simulink model "amalifuzzypid"  (R2021a)
settings: Solver=FixedStepAuto  StartTime=0.0  StopTime=20  RelTol=1e-2  EnableMultiTasking=on
InitFcn:
  | Ts=0.01;
  | 
  | Kpmin1 = 0.1;
  | Kpmax1 = 5;
  | Kdmin1 = 0;
  | Kdmax1 = 2;
undefined symbols (not defined in the file): DiscIntNeverNeededParam
libraries: raspberrypiCommlib x6, pid_lib x4, raspberrypiBasiclib x4, fuzblock x2
settings Model: Creator=pouria  LastModifiedBy=pouria
settings SolverCC: AlgebraicLoopSolver=TrustRegion  PositivePriorityOrder=on
settings DataIOCC: LimitDataPoints=on  SaveFormat=Array  ReturnWorkspaceOutputs=off
settings OptimizationCC: EnhancedBackFolding=on  PassReuseOutputArgsAs=Individual arguments  ZeroExternalMemoryAtStartup=off  ZeroInternalMemoryAtStartup=off  MaxStackSize=64  OptimizeBlockOrder=speed  DifferentSizesBufferReuse=on  OptimizationCustomize=off  EfficientTunableParamExpr=on
settings DebuggingCC: ParameterTunabilityLossMsg=error  SFUnexpectedBacktrackingDiag=warning  SFNoUnconditionalDefaultTransitionDiag=warning  SFExecutionAtInitializationDiag=none  SFMachineParentedDataDiag=warning  ArithmeticOperatorsInVariantConditions=warning
settings HardwareCC: ProdBitPerPointer=32  ProdBitPerSizeT=32  ProdBitPerPtrDiffT=32  ProdLargestAtomicInteger=Long  ProdLargestAtomicFloat=Double  ProdWordSize=32  ProdLongLongMode=on  ProdHWDeviceType=ARM Compatible->ARM Cortex
settings ModelReferenceCC: PropagateSignalLabelsOutOfModel=off
settings SFSimCC: SimUseLocalCustomCode=off  CustomCodeUndefinedFunction=UseInterfaceOnly
settings RTWCC: SystemTargetFile=ert.tlc  HardwareBoard=Raspberry Pi  TLCOptions="-aInlineSetEventsForThisBaseRateFcn=TLC_FALSE -aSuppressMultiTaskScheduler=TLC_FALSE  -aRateBasedStepFcn=0"  TemplateMakefile=ert_default_tmf  RTWUseLocalCustomCode=off  Toolchain=GNU GCC Embedded Linux  BuildConfiguration=Faster Runs
settings CodeAppCC: ForceParamTrailComments=on  IgnoreCustomStorageClasses=off  OperatorAnnotations=on  SimulinkDataObjDesc=on  SFDataObjDesc=on  InsertBlockDesc=on
settings ERTTargetCC: SupportContinuousTime=on  SupportVariableSizeSignals=on  ExtModeTransport=2  ExtModeStaticAlloc=on  ExtModeMexFile=ext_xcp  ExtModeIntrfLevel=Level2 - Open
settings ConfigComp: CovMetricSettings=dw  CovSaveCumulativeToWorkspaceVar=on  CovSaveSingleToWorkspaceVar=on  CovExternalEMLEnable=off  CovSFcnEnable=off

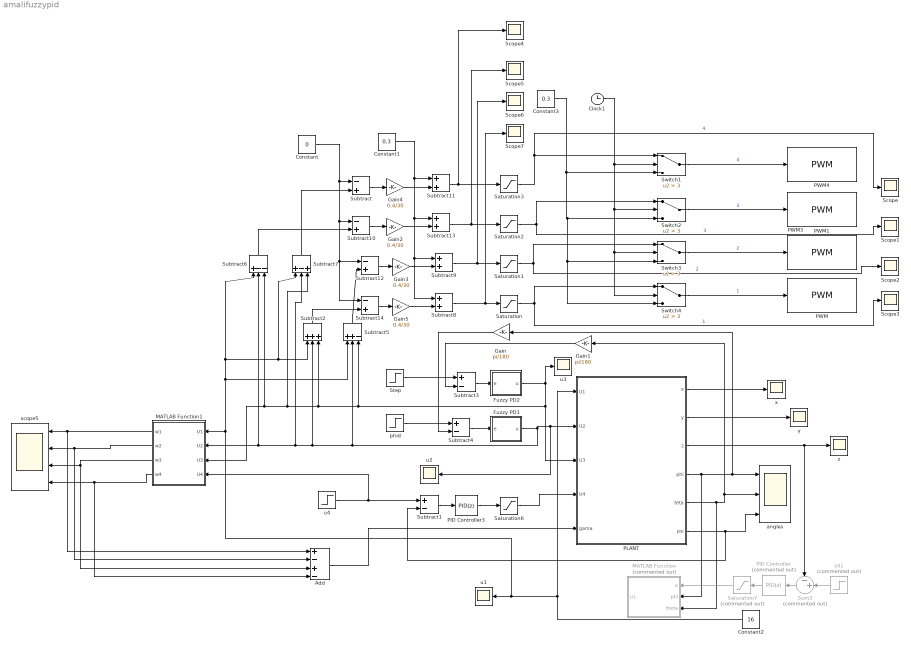
== system amalifuzzypid ==
  Add : Sum  Inputs=+-+-
  Clock1 : Clock
  Constant : Constant  Value=0  SampleTime=Ts
  Constant1 : Constant  Value=0.3  SampleTime=Ts
  Constant2 : Constant  Value=16  SampleTime=Ts
  Constant3 : Constant  Value=0.3  SampleTime=Ts
  Fuzzy PD1 : Subsystem
  Fuzzy PD2 : Subsystem
  Gain : Gain  Gain=pi/180
  Gain1 : Gain  Gain=pi/180
  Gain{2..5} (4 alike) : Gain  Gain=0.4/30
  MATLAB Function : MATLAB Function  Commented=on  TreatAsAtomicUnit=on
  MATLAB Function1 : MATLAB Function  TreatAsAtomicUnit=on
  PID Controller : pid_lib/PID Controller  Commented=on  Controller=PID  Form=Parallel  TimeDomain=Discrete-time  UseExternalTs=off  SampleTime=0.01  IntegratorMethod=Forward Euler  FilterMethod=Forward Euler  ControllerParametersSource=internal  P=5  I=2  D=15  UseFilter=on  N=20  TunerSelectOption=Transfer Function Based (PID Tuner App)  InitialConditionSource=internal  InitialConditionForIntegrator=0  InitialConditionForFilter=0  DifferentiatorICPrevScaledInput=0  ExternalReset=none  TrackingMode=off  Kt=1  LimitOutput=off  SatLimitsSource=internal  UpperSaturationLimit=inf  LowerSaturationLimit=-inf  LinearizeAsGain=on  AntiWindupMode=none  Kb=1  POutMin=[]  POutMax=[]  IOutMin=[]  IOutMax=[]  DOutMin=[]  DOutMax=[]  NOutMin=[]  NOutMax=[]  SumOutMin=[]  SumOutMax=[]  SaturationOutMin=[]  SaturationOutMax=[]  PParamMin=[]  PParamMax=[]  IParamMin=[]  IParamMax=[]  DParamMin=[]  DParamMax=[]  NParamMin=[]  NParamMax=[]  KbParamMin=[]  KbParamMax=[]  KtParamMin=[]  KtParamMax=[]  KbOutMin=[]  KbOutMax=[]  KtOutMin=[]  KtOutMax=[]  IntegratorOutMin=[]  IntegratorOutMax=[]  FilterOutMin=[]  FilterOutMax=[]  SumI1OutMin=[]  SumI1OutMax=[]  SumI2OutMin=[]  SumI2OutMax=[]  SumI3OutMin=[]  SumI3OutMax=[]  SumI4OutMin=[]  SumI4OutMax=[]  SumDOutMin=[]  SumDOutMax=[]  DifferentiatorOutMin=[]  DifferentiatorOutMax=[]  FilterDiffOutCoefMin=[]  FilterDiffOutCoefMax=[]  ReciprocalOutMin=[]  ReciprocalOutMax=[]  SumDenOutMin=[]  SumDenOutMax=[]  SumNumOutMin=[]  SumNumOutMax=[]  DivideOutMin=[]  DivideOutMax=[]  UdiffTsProdOutMin=[]  UdiffTsProdOutMax=[]  NTsProdOutMin=[]  NTsProdOutMax=[]  UintegralTsProdOutMin=[]  UintegralTsProdOutMax=[]  UngainTsProdOutMin=[]  UngainTsProdOutMax=[]  IntegratorContinuousStateAttributes=''  IntegratorStateMustResolveToSignalObject=off  IntegratorRTWStateStorageClass=Auto  FilterContinuousStateAttributes=''  FilterStateMustResolveToSignalObject=off  FilterRTWStateStorageClass=Auto  ParallelPVariant=InternalParameters  IdealPVariant=Disabled  IVariant=InternalParameters  DVariant=InternalParameters  IntegratorVariant=Discrete  SatVariant=Disabled  AWVariant=Passthrough  PCopyVariant=Disabled  TRVariant=Disabled  FdbkBlocksVariant=Forward  IdealPFdbkVariant=Disabled  SatFdbkVariant=Disabled  DerivativeFilterVariant=ForwardEulerFilter  NVariant=InternalParameters  NCopyVariant=Disabled  FilterICVariant=InternalICsFilter  IntegratorICVariant=InternalICs  ExternalResetVariant=Disabled  TRSumVariant=Passthrough  SumFdbkVariant=Disabled  SumVariant=Sum_PID  TsampFilterVariant=InternalTs  TsampNgainVariant=Passthrough  TsampIntegralVariant=Passthrough  ExternalSaturationOutDataTypeStr=Inherit: Same as second input
  PID Controller3 : pid_lib/PID Controller  Controller=PID  Form=Parallel  TimeDomain=Discrete-time  UseExternalTs=off  SampleTime=Ts  IntegratorMethod=Forward Euler  FilterMethod=Forward Euler  ControllerParametersSource=internal  P=0  I=0  D=0  UseFilter=on  N=20  TunerSelectOption=Transfer Function Based (PID Tuner App)  InitialConditionSource=internal  InitialConditionForIntegrator=0  InitialConditionForFilter=0  DifferentiatorICPrevScaledInput=0  ExternalReset=none  TrackingMode=off  Kt=1  LimitOutput=off  SatLimitsSource=internal  UpperSaturationLimit=inf  LowerSaturationLimit=-inf  LinearizeAsGain=on  AntiWindupMode=none  Kb=1  POutMin=[]  POutMax=[]  IOutMin=[]  IOutMax=[]  DOutMin=[]  DOutMax=[]  NOutMin=[]  NOutMax=[]  SumOutMin=[]  SumOutMax=[]  SaturationOutMin=[]  SaturationOutMax=[]  PParamMin=[]  PParamMax=[]  IParamMin=[]  IParamMax=[]  DParamMin=[]  DParamMax=[]  NParamMin=[]  NParamMax=[]  KbParamMin=[]  KbParamMax=[]  KtParamMin=[]  KtParamMax=[]  KbOutMin=[]  KbOutMax=[]  KtOutMin=[]  KtOutMax=[]  IntegratorOutMin=[]  IntegratorOutMax=[]  FilterOutMin=[]  FilterOutMax=[]  SumI1OutMin=[]  SumI1OutMax=[]  SumI2OutMin=[]  SumI2OutMax=[]  SumI3OutMin=[]  SumI3OutMax=[]  SumI4OutMin=[]  SumI4OutMax=[]  SumDOutMin=[]  SumDOutMax=[]  DifferentiatorOutMin=[]  DifferentiatorOutMax=[]  FilterDiffOutCoefMin=[]  FilterDiffOutCoefMax=[]  ReciprocalOutMin=[]  ReciprocalOutMax=[]  SumDenOutMin=[]  SumDenOutMax=[]  SumNumOutMin=[]  SumNumOutMax=[]  DivideOutMin=[]  DivideOutMax=[]  UdiffTsProdOutMin=[]  UdiffTsProdOutMax=[]  NTsProdOutMin=[]  NTsProdOutMax=[]  UintegralTsProdOutMin=[]  UintegralTsProdOutMax=[]  UngainTsProdOutMin=[]  UngainTsProdOutMax=[]  IntegratorContinuousStateAttributes=''  IntegratorStateMustResolveToSignalObject=off  IntegratorRTWStateStorageClass=Auto  FilterContinuousStateAttributes=''  FilterStateMustResolveToSignalObject=off  FilterRTWStateStorageClass=Auto  ParallelPVariant=InternalParameters  IdealPVariant=Disabled  IVariant=InternalParameters  DVariant=InternalParameters  IntegratorVariant=Discrete  SatVariant=Disabled  AWVariant=Passthrough  PCopyVariant=Disabled  TRVariant=Disabled  FdbkBlocksVariant=Forward  IdealPFdbkVariant=Disabled  SatFdbkVariant=Disabled  DerivativeFilterVariant=ForwardEulerFilter  NVariant=InternalParameters  NCopyVariant=Disabled  FilterICVariant=InternalICsFilter  IntegratorICVariant=InternalICs  ExternalResetVariant=Disabled  TRSumVariant=Passthrough  SumFdbkVariant=Disabled  SumVariant=Sum_PID  TsampFilterVariant=InternalTs  TsampNgainVariant=Passthrough  TsampIntegralVariant=Passthrough  ExternalSaturationOutDataTypeStr=Inherit: Same as second input
  PLANT : Subsystem
  PWM : raspberrypiBasiclib/PWM  board=Pi 3 Model B+  Pin_=21  Frequency=400  blockPlatform=Raspberry Pi
      settings: SourceProductBaseCode=RASPPI
  PWM1 : raspberrypiBasiclib/PWM  board=Pi 3 Model B+  Pin_=20  Frequency=400  blockPlatform=Raspberry Pi
      settings: SourceProductBaseCode=RASPPI
  PWM3 : raspberrypiBasiclib/PWM  board=Pi 3 Model B+  Pin_=16  Frequency=400  blockPlatform=Raspberry Pi
      settings: SourceProductBaseCode=RASPPI
  PWM4 : raspberrypiBasiclib/PWM  board=Pi 3 Model B+  Pin_=19  Frequency=400  blockPlatform=Raspberry Pi
      settings: SourceProductBaseCode=RASPPI
  Saturation{,1..3} (4 alike) : Saturate  UpperLimit=0.63  LowerLimit=0.3
  Saturation6 : Saturate
  Saturation7 : Saturate  Commented=on  UpperLimit=10  LowerLimit=-10
  Scope{,1..7} (8 alike) : Scope
  Step : Step  Time=0  After=0  SampleTime=0
  Subtract{,10,12,14} (4 alike) : Sum  Inputs=-+
  Subtract1 : Sum  Inputs=+-
  Subtract{8..9,11,13} (4 alike) : Sum
  Subtract2 : Sum  Inputs=+++
  Subtract3 : Sum  Inputs=+-
  Subtract4 : Sum  Inputs=+-
  Subtract5 : Sum  Inputs=++-
  Subtract6 : Sum  Inputs=+--
  Subtract7 : Sum  Inputs=+-+
  Sum2 : Sum  Commented=on  Inputs=-+|
  Switch{1..4} (4 alike) : Switch  Criteria=u2 > Threshold  Threshold=3
  angles : Scope  NumInputPorts=3
  phid : Step  Time=0  After=0  SampleTime=Ts
  scope5 : Scope  NumInputPorts=4
  u1 : Scope
  u2 : Scope
  u3 : Scope
  u4 : Step  Time=0  After=0  SampleTime=Ts
  x : Scope
  y : Scope
  z : Scope
  zd1 : Step  Commented=on  Time=0  After=0  SampleTime=0
  wires:
  PLANT/6(psi) -> angles/3, Subtract1/2
  PLANT/1(x) -> x/1
  PLANT/2(y) -> y/1
  Subtract4/1 -> Fuzzy PD1/1(e)
  Subtract3/1 -> Fuzzy PD2/1(e)
  Add/1 -> PLANT/5(gama)
  MATLAB Function1/1(w1) -> Add/1, scope5/1
  MATLAB Function1/3(w3) -> Add/3, scope5/3
  MATLAB Function1/4(w4) -> scope5/4, Add/4
  phid/1 -> Subtract4/1
  u4/1 -> MATLAB Function1/4(U4), Subtract1/1
  Subtract1/1 -> PID Controller3/1
  PID Controller3/1 -> Saturation6/1
  MATLAB Function1/2(w2) -> Add/2, scope5/2
  zd1/1 -> Sum2/2
  PLANT/3(z) -> z/1, Sum2/1
  PLANT/4(phi) -> MATLAB Function/2(phi), angles/1, Gain/1
  PID Controller/1 -> Saturation7/1
  PLANT/5(teta) -> MATLAB Function/3(theta), angles/2, Gain1/1
  Sum2/1 -> PID Controller/1
  Saturation/1 -> Switch4/1, Scope3/1  "1"
  Saturation1/1 -> Switch3/1, Scope2/1  "2"
  Saturation2/1 -> Switch2/1, Scope1/1  "3"
  Saturation3/1 -> Switch1/1, Scope/1  "4"
  Gain/1 -> Subtract4/2
  Gain1/1 -> Subtract3/2
  Fuzzy PD2/1(u) -> PLANT/3(U3), Subtract5/3, Subtract2/3, Subtract6/3, MATLAB Function1/3(U3), Subtract7/3, u3/1
  Saturation6/1 -> PLANT/4(U4)
  Constant2/1 -> MATLAB Function1/1(U1), Subtract5/1, Subtract2/1, Subtract7/1, Subtract6/1, u1/1, PLANT/1(U1)
  Subtract7/1 -> Subtract/2
  Subtract6/1 -> Subtract10/2
  Subtract5/1 -> Subtract12/2
  Constant/1 -> Subtract14/1, Subtract12/1, Subtract10/1, Subtract/1
  Subtract2/1 -> Subtract14/2
  Saturation7/1 -> MATLAB Function/1(e)
  Fuzzy PD1/1(u) -> u2/1, PLANT/2(U2), Subtract7/2, Subtract6/2, MATLAB Function1/2(U2), Subtract2/2, Subtract5/2
  Clock1/1 -> Switch4/2, Switch3/2, Switch2/2, Switch1/2
  Switch1/1 -> PWM4/1  "4"
  Constant3/1 -> Switch1/3, Switch3/3, Switch4/3, Switch2/3
  Switch2/1 -> PWM1/1  "3"
  Switch3/1 -> PWM3/1  "2"
  Switch4/1 -> PWM/1  "1"
  Subtract9/1 -> Scope6/1, Saturation1/1
  Subtract13/1 -> Scope5/1, Saturation2/1
  Subtract11/1 -> Scope4/1, Saturation3/1
  Subtract8/1 -> Scope7/1, Saturation/1
  Subtract14/1 -> Gain5/1
  Subtract12/1 -> Gain3/1
  Subtract10/1 -> Gain2/1
  Subtract/1 -> Gain4/1
  Constant1/1 -> Subtract8/1, Subtract9/1, Subtract13/1, Subtract11/1
  Gain4/1 -> Subtract11/2
  Gain2/1 -> Subtract13/2
  Gain3/1 -> Subtract9/2
  Gain5/1 -> Subtract8/2
  Step/1 -> Subtract3/1

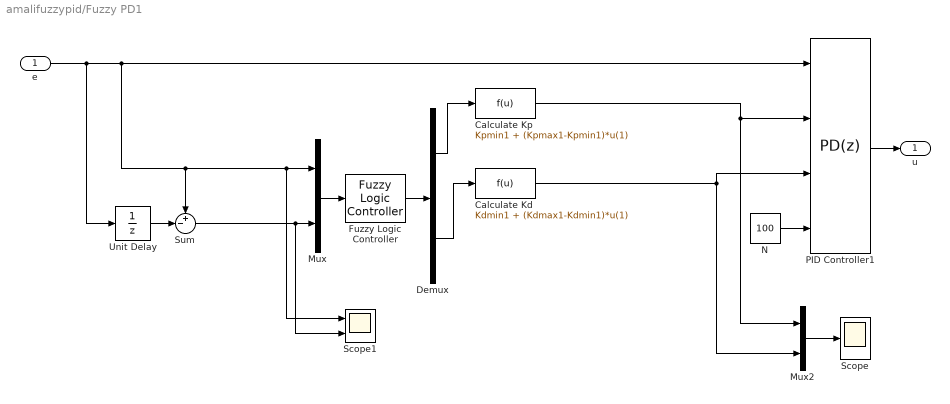
== system amalifuzzypid/Fuzzy PD1 ==
  e : Inport
  Calculate Kd : Fcn  Expr=Kdmin1 + (Kdmax1-Kdmin1)*u(1)
  Calculate Kp : Fcn  Expr=Kpmin1 + (Kpmax1-Kpmin1)*u(1)
  Demux : Demux  Outputs=2
  Fuzzy Logic Controller : fuzblock/Fuzzy Logic  Controller  FIS='fuzzy_pd1.fis'  OutputSampleNumber=101  DataType=double  FuzzifiedInputs=off  RuleFiringStrengths=off  RuleOutputs=off  AggregatedOutputs=off  SimulateUsing=Interpreted execution  OutOfRangeInputValueMessage=warning  NoRuleFiredMessage=warning  EmptyOutputFuzzySetMessage=warning
  Mux : Mux  Inputs=2
  Mux2 : Mux  Inputs=2
  N : Constant  Value=100  SampleTime=Ts
  PID Controller1 : pid_lib/PID Controller  Controller=PD  Form=Parallel  TimeDomain=Discrete-time  UseExternalTs=off  SampleTime=Ts  IntegratorMethod=Forward Euler  FilterMethod=Forward Euler  ControllerParametersSource=external  P=0.6*4.6737  I=1.2*4.6737/3.26  D=0.6*4.6737*3.26/8  UseFilter=on  N=100  TunerSelectOption=Transfer Function Based (PID Tuner App)  InitialConditionSource=internal  InitialConditionForIntegrator=0  InitialConditionForFilter=0  DifferentiatorICPrevScaledInput=0  ExternalReset=none  TrackingMode=off  Kt=1  LimitOutput=off  SatLimitsSource=internal  UpperSaturationLimit=inf  LowerSaturationLimit=-inf  LinearizeAsGain=on  AntiWindupMode=none  Kb=1  POutMin=[]  POutMax=[]  IOutMin=[]  IOutMax=[]  DOutMin=[]  DOutMax=[]  NOutMin=[]  NOutMax=[]  SumOutMin=[]  SumOutMax=[]  SaturationOutMin=[]  SaturationOutMax=[]  PParamMin=[]  PParamMax=[]  IParamMin=[]  IParamMax=[]  DParamMin=[]  DParamMax=[]  NParamMin=[]  NParamMax=[]  KbParamMin=[]  KbParamMax=[]  KtParamMin=[]  KtParamMax=[]  KbOutMin=[]  KbOutMax=[]  KtOutMin=[]  KtOutMax=[]  IntegratorOutMin=[]  IntegratorOutMax=[]  FilterOutMin=[]  FilterOutMax=[]  SumI1OutMin=[]  SumI1OutMax=[]  SumI2OutMin=[]  SumI2OutMax=[]  SumI3OutMin=[]  SumI3OutMax=[]  SumI4OutMin=[]  SumI4OutMax=[]  SumDOutMin=[]  SumDOutMax=[]  DifferentiatorOutMin=[]  DifferentiatorOutMax=[]  FilterDiffOutCoefMin=[]  FilterDiffOutCoefMax=[]  ReciprocalOutMin=[]  ReciprocalOutMax=[]  SumDenOutMin=[]  SumDenOutMax=[]  SumNumOutMin=[]  SumNumOutMax=[]  DivideOutMin=[]  DivideOutMax=[]  UdiffTsProdOutMin=[]  UdiffTsProdOutMax=[]  NTsProdOutMin=[]  NTsProdOutMax=[]  UintegralTsProdOutMin=[]  UintegralTsProdOutMax=[]  UngainTsProdOutMin=[]  UngainTsProdOutMax=[]  IntegratorContinuousStateAttributes=''  IntegratorStateMustResolveToSignalObject=off  IntegratorRTWStateStorageClass=Auto  FilterContinuousStateAttributes=''  FilterStateMustResolveToSignalObject=off  FilterRTWStateStorageClass=Auto  ParallelPVariant=ExternalParameters  IdealPVariant=Disabled  IVariant=Disabled  DVariant=ExternalParameters  IntegratorVariant=Disabled  SatVariant=Disabled  AWVariant=Disabled  PCopyVariant=Disabled  TRVariant=Disabled  FdbkBlocksVariant=Forward  IdealPFdbkVariant=Disabled  SatFdbkVariant=Disabled  DerivativeFilterVariant=ForwardEulerFilter  NVariant=ExternalParameters  NCopyVariant=Disabled  FilterICVariant=InternalICsFilter  IntegratorICVariant=Disabled  ExternalResetVariant=Disabled  TRSumVariant=Passthrough  SumFdbkVariant=Disabled  SumVariant=Sum_PD  TsampFilterVariant=InternalTs  TsampNgainVariant=Passthrough  TsampIntegralVariant=Disabled_SignalSpec  ExternalSaturationOutDataTypeStr=Inherit: Same as second input
  Scope : Scope
  Scope1 : Scope  NumInputPorts=2
  Sum : Sum  Inputs=+-|
  Unit Delay : UnitDelay  SampleTime=Ts  HasFrameUpgradeWarning=on
  u : Outport
  wires:
  PID Controller1/1 -> u/1
  N/1 -> PID Controller1/4
  Mux/1 -> Fuzzy Logic Controller/1
  Fuzzy Logic Controller/1 -> Demux/1
  Demux/1 -> Calculate Kp/1
  Calculate Kp/1 -> Mux2/1, PID Controller1/2
  Demux/2 -> Calculate Kd/1
  Calculate Kd/1 -> Mux2/2, PID Controller1/3
  Unit Delay/1 -> Sum/2
  Mux2/1 -> Scope/1
  e/1 -> Mux/1, Scope1/1, Sum/1, PID Controller1/1, Unit Delay/1
  Sum/1 -> Scope1/2, Mux/2

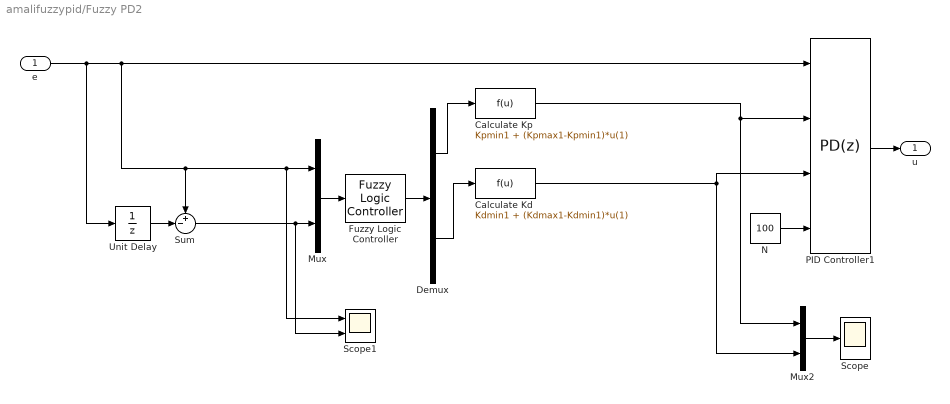
== system amalifuzzypid/Fuzzy PD2 ==
  e : Inport
  Calculate Kd : Fcn  Expr=Kdmin1 + (Kdmax1-Kdmin1)*u(1)
  Calculate Kp : Fcn  Expr=Kpmin1 + (Kpmax1-Kpmin1)*u(1)
  Demux : Demux  Outputs=2
  Fuzzy Logic Controller : fuzblock/Fuzzy Logic  Controller  FIS='fuzzy_pd1.fis'  OutputSampleNumber=101  DataType=double  FuzzifiedInputs=off  RuleFiringStrengths=off  RuleOutputs=off  AggregatedOutputs=off  SimulateUsing=Interpreted execution  OutOfRangeInputValueMessage=warning  NoRuleFiredMessage=warning  EmptyOutputFuzzySetMessage=warning
  Mux : Mux  Inputs=2
  Mux2 : Mux  Inputs=2
  N : Constant  Value=100  SampleTime=Ts
  PID Controller1 : pid_lib/PID Controller  Controller=PD  Form=Parallel  TimeDomain=Discrete-time  UseExternalTs=off  SampleTime=Ts  IntegratorMethod=Forward Euler  FilterMethod=Forward Euler  ControllerParametersSource=external  P=0.6*4.6737  I=1.2*4.6737/3.26  D=0.6*4.6737*3.26/8  UseFilter=on  N=100  TunerSelectOption=Transfer Function Based (PID Tuner App)  InitialConditionSource=internal  InitialConditionForIntegrator=0  InitialConditionForFilter=0  DifferentiatorICPrevScaledInput=0  ExternalReset=none  TrackingMode=off  Kt=1  LimitOutput=off  SatLimitsSource=internal  UpperSaturationLimit=inf  LowerSaturationLimit=-inf  LinearizeAsGain=on  AntiWindupMode=none  Kb=1  POutMin=[]  POutMax=[]  IOutMin=[]  IOutMax=[]  DOutMin=[]  DOutMax=[]  NOutMin=[]  NOutMax=[]  SumOutMin=[]  SumOutMax=[]  SaturationOutMin=[]  SaturationOutMax=[]  PParamMin=[]  PParamMax=[]  IParamMin=[]  IParamMax=[]  DParamMin=[]  DParamMax=[]  NParamMin=[]  NParamMax=[]  KbParamMin=[]  KbParamMax=[]  KtParamMin=[]  KtParamMax=[]  KbOutMin=[]  KbOutMax=[]  KtOutMin=[]  KtOutMax=[]  IntegratorOutMin=[]  IntegratorOutMax=[]  FilterOutMin=[]  FilterOutMax=[]  SumI1OutMin=[]  SumI1OutMax=[]  SumI2OutMin=[]  SumI2OutMax=[]  SumI3OutMin=[]  SumI3OutMax=[]  SumI4OutMin=[]  SumI4OutMax=[]  SumDOutMin=[]  SumDOutMax=[]  DifferentiatorOutMin=[]  DifferentiatorOutMax=[]  FilterDiffOutCoefMin=[]  FilterDiffOutCoefMax=[]  ReciprocalOutMin=[]  ReciprocalOutMax=[]  SumDenOutMin=[]  SumDenOutMax=[]  SumNumOutMin=[]  SumNumOutMax=[]  DivideOutMin=[]  DivideOutMax=[]  UdiffTsProdOutMin=[]  UdiffTsProdOutMax=[]  NTsProdOutMin=[]  NTsProdOutMax=[]  UintegralTsProdOutMin=[]  UintegralTsProdOutMax=[]  UngainTsProdOutMin=[]  UngainTsProdOutMax=[]  IntegratorContinuousStateAttributes=''  IntegratorStateMustResolveToSignalObject=off  IntegratorRTWStateStorageClass=Auto  FilterContinuousStateAttributes=''  FilterStateMustResolveToSignalObject=off  FilterRTWStateStorageClass=Auto  ParallelPVariant=ExternalParameters  IdealPVariant=Disabled  IVariant=Disabled  DVariant=ExternalParameters  IntegratorVariant=Disabled  SatVariant=Disabled  AWVariant=Disabled  PCopyVariant=Disabled  TRVariant=Disabled  FdbkBlocksVariant=Forward  IdealPFdbkVariant=Disabled  SatFdbkVariant=Disabled  DerivativeFilterVariant=ForwardEulerFilter  NVariant=ExternalParameters  NCopyVariant=Disabled  FilterICVariant=InternalICsFilter  IntegratorICVariant=Disabled  ExternalResetVariant=Disabled  TRSumVariant=Passthrough  SumFdbkVariant=Disabled  SumVariant=Sum_PD  TsampFilterVariant=InternalTs  TsampNgainVariant=Passthrough  TsampIntegralVariant=Disabled_SignalSpec  ExternalSaturationOutDataTypeStr=Inherit: Same as second input
  Scope : Scope
  Scope1 : Scope  NumInputPorts=2
  Sum : Sum  Inputs=+-|
  Unit Delay : UnitDelay  SampleTime=Ts  HasFrameUpgradeWarning=on
  u : Outport
  wires:
  PID Controller1/1 -> u/1
  N/1 -> PID Controller1/4
  Mux/1 -> Fuzzy Logic Controller/1
  Fuzzy Logic Controller/1 -> Demux/1
  Demux/1 -> Calculate Kp/1
  Calculate Kp/1 -> Mux2/1, PID Controller1/2
  Demux/2 -> Calculate Kd/1
  Calculate Kd/1 -> Mux2/2, PID Controller1/3
  Unit Delay/1 -> Sum/2
  Mux2/1 -> Scope/1
  e/1 -> Mux/1, Scope1/1, Sum/1, PID Controller1/1, Unit Delay/1
  Sum/1 -> Scope1/2, Mux/2

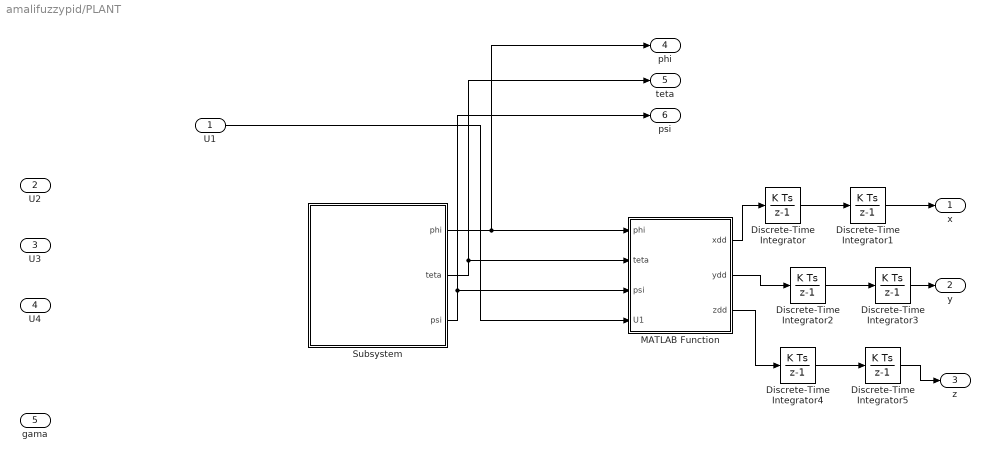
== system amalifuzzypid/PLANT ==
  U1 : Inport
  U2 : Inport  Port=2
  U3 : Inport  Port=3
  U4 : Inport  Port=4
  gama : Inport  Port=5
  Discrete-Time Integrator{,1..5} (6 alike) : DiscreteIntegrator  SampleTime=Ts  ICPrevOutput=DiscIntNeverNeededParam  ICPrevScaledInput=DiscIntNeverNeededParam
  MATLAB Function : MATLAB Function  TreatAsAtomicUnit=on
  Subsystem : Subsystem
  x : Outport
  y : Outport  Port=2
  z : Outport  Port=3
  phi : Outport  Port=4
  teta : Outport  Port=5
  psi : Outport  Port=6
  wires:
  Discrete-Time Integrator1/1 -> x/1
  MATLAB Function/1(xdd) -> Discrete-Time Integrator/1
  U1/1 -> MATLAB Function/4(U1)
  Discrete-Time Integrator/1 -> Discrete-Time Integrator1/1
  Discrete-Time Integrator2/1 -> Discrete-Time Integrator3/1
  Discrete-Time Integrator3/1 -> y/1
  MATLAB Function/2(ydd) -> Discrete-Time Integrator2/1
  Discrete-Time Integrator4/1 -> Discrete-Time Integrator5/1
  Discrete-Time Integrator5/1 -> z/1
  MATLAB Function/3(zdd) -> Discrete-Time Integrator4/1
  Subsystem/1(phi) -> phi/1, MATLAB Function/1(phi)
  Subsystem/2(teta) -> teta/1, MATLAB Function/2(teta)
  Subsystem/3(psi) -> psi/1, MATLAB Function/3(psi)

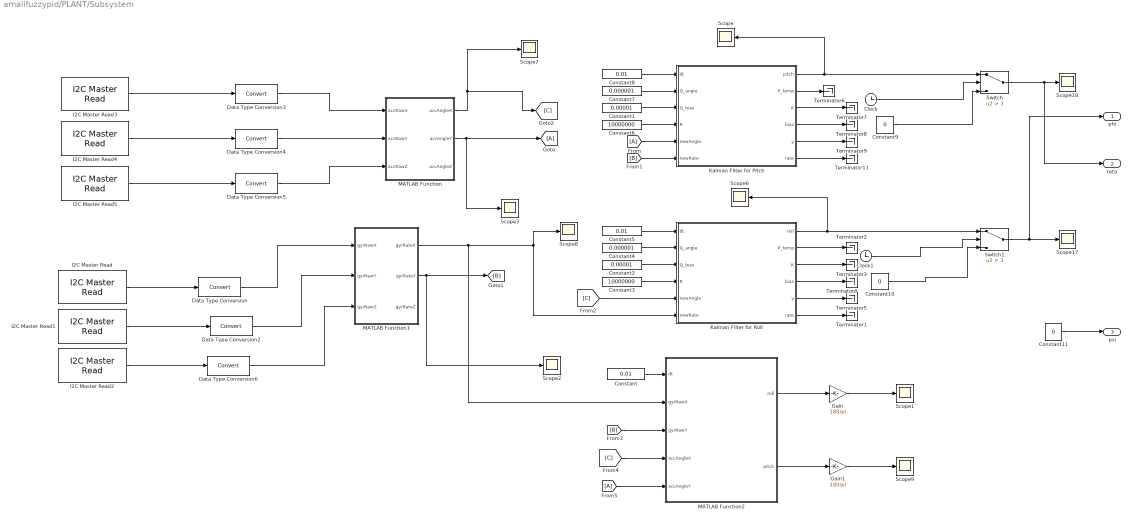
== system amalifuzzypid/PLANT/Subsystem ==
  Clock : Clock
  Clock1 : Clock
  Constant : Constant  Value=0.01
  Constant1 : Constant  Value=0.00001  SampleTime=0.01
  Constant10 : Constant  Value=0  SampleTime=Ts
  Constant11 : Constant  Value=0  SampleTime=Ts
  Constant2 : Constant  Value=0.00001  SampleTime=0.01
  Constant3 : Constant  Value=10000000  SampleTime=0.01
  Constant4 : Constant  Value=0.000001  SampleTime=0.01
  Constant5 : Constant  Value=0.01  SampleTime=0.01
  Constant6 : Constant  Value=10000000  SampleTime=0.01
  Constant7 : Constant  Value=0.000001  SampleTime=0.01
  Constant8 : Constant  Value=0.01  SampleTime=0.01
  Constant9 : Constant  Value=0  SampleTime=Ts
  Data Type Conversion{,2..6} (6 alike) : DataTypeConversion
  Gain : Gain  Gain=180/pi
  Gain1 : Gain  Gain=180/pi
  I2C Master Read : raspberrypiCommlib/I2C Master Read  BoardProperty=Pi 3 Model B+  Mode=Master  SlaveAddress="hex2dec(\"0x68\")"  SlaveByteOrder=BigEndian  Direction=Receiver  RegisterAddressMode=on  RegisterAddress=67  SlaveDataType=int16  DataLength=1  NoAck=off  RepeatedStart=off  OutputStatus=off  SampleTime=0.01
      settings: SourceProductBaseCode=RASPPI
  I2C Master Read1 : raspberrypiCommlib/I2C Master Read  BoardProperty=Pi 3 Model B+  Mode=Master  SlaveAddress="hex2dec(\"0x68\")"  SlaveByteOrder=BigEndian  Direction=Receiver  RegisterAddressMode=on  RegisterAddress=69  SlaveDataType=int16  DataLength=1  NoAck=off  RepeatedStart=off  OutputStatus=off  SampleTime=0.01
      settings: SourceProductBaseCode=RASPPI
  I2C Master Read2 : raspberrypiCommlib/I2C Master Read  BoardProperty=Pi 3 Model B+  Mode=Master  SlaveAddress="hex2dec(\"0x68\")"  SlaveByteOrder=BigEndian  Direction=Receiver  RegisterAddressMode=on  RegisterAddress=71  SlaveDataType=int16  DataLength=1  NoAck=off  RepeatedStart=off  OutputStatus=off  SampleTime=0.01
      settings: SourceProductBaseCode=RASPPI
  I2C Master Read3 : raspberrypiCommlib/I2C Master Read  BoardProperty=Pi 3 Model B+  Mode=Master  SlaveAddress="hex2dec(\"0x68\")"  SlaveByteOrder=BigEndian  Direction=Receiver  RegisterAddressMode=on  RegisterAddress=59  SlaveDataType=int16  DataLength=1  NoAck=off  RepeatedStart=off  OutputStatus=off  SampleTime=0.01
      settings: SourceProductBaseCode=RASPPI
  I2C Master Read4 : raspberrypiCommlib/I2C Master Read  BoardProperty=Pi 3 Model B+  Mode=Master  SlaveAddress="hex2dec(\"0x68\")"  SlaveByteOrder=BigEndian  Direction=Receiver  RegisterAddressMode=on  RegisterAddress=61  SlaveDataType=int16  DataLength=1  NoAck=off  RepeatedStart=off  OutputStatus=off  SampleTime=0.01
      settings: SourceProductBaseCode=RASPPI
  I2C Master Read5 : raspberrypiCommlib/I2C Master Read  BoardProperty=Pi 3 Model B+  Mode=Master  SlaveAddress="hex2dec(\"0x68\")"  SlaveByteOrder=BigEndian  Direction=Receiver  RegisterAddressMode=on  RegisterAddress=63  SlaveDataType=int16  DataLength=1  NoAck=off  RepeatedStart=off  OutputStatus=off  SampleTime=0.01
      settings: SourceProductBaseCode=RASPPI
  Kalman Filter for Pitch : MATLAB Function  TreatAsAtomicUnit=on
  Kalman Filter for Roll : MATLAB Function  TreatAsAtomicUnit=on
  MATLAB Function : MATLAB Function  TreatAsAtomicUnit=on
  MATLAB Function1 : MATLAB Function  TreatAsAtomicUnit=on
  MATLAB Function2 : MATLAB Function  TreatAsAtomicUnit=on
  Scope{,1..3,6..9,17..18} (10 alike) : Scope
  Switch : Switch  Criteria=u2 > Threshold  Threshold=3
  Switch1 : Switch  Criteria=u2 > Threshold  Threshold=3
  Terminator{1..9,11} (10 alike) : Terminator
  phi : Outport
  teta : Outport  Port=2
  psi : Outport  Port=3
  wires:
  Constant/1 -> MATLAB Function2/1(dt)
  Clock/1 -> Switch/2
  Gain1/1 -> Scope9/1
  I2C Master Read1/1 -> Data Type Conversion2/1
  Gain/1 -> Scope1/1
  [A] -> MATLAB Function2/5(accAngleY)
  Switch/1 -> teta/1, Scope18/1
  [B] -> MATLAB Function2/3(gyrRawY)
  Constant3/1 -> Kalman Filter for Roll/4(R)
  MATLAB Function/2(accAngleY) -> [A], Scope3/1
  Data Type Conversion6/1 -> MATLAB Function1/3(gyrRawZ)
  Switch1/1 -> phi/1, Scope17/1
  MATLAB Function2/2(pitch) -> Gain1/1
  MATLAB Function/1(accAngleX) -> [C], Scope7/1
  Kalman Filter for Pitch/1(pitch) -> Switch/1, Scope/1
  Constant9/1 -> Switch/3
  Kalman Filter for Roll/1(roll) -> Switch1/1, Scope6/1
  Kalman Filter for Roll/3(K) -> Terminator3/1
  Clock1/1 -> Switch1/2
  I2C Master Read/1 -> Data Type Conversion/1
  Constant10/1 -> Switch1/3
  Data Type Conversion3/1 -> MATLAB Function/1(accRawX)
  Constant5/1 -> Kalman Filter for Roll/1(dt)
  I2C Master Read2/1 -> Data Type Conversion6/1
  MATLAB Function1/1(gyrRateX) -> MATLAB Function2/2(gyrRawX), Kalman Filter for Roll/6(newRate), Scope8/1
  [C] -> MATLAB Function2/4(accAngleX)
  Kalman Filter for Roll/4(bias) -> Terminator4/1
  Kalman Filter for Pitch/5(y) -> Terminator9/1
  Kalman Filter for Pitch/3(K) -> Terminator7/1
  Kalman Filter for Pitch/2(P_temp) -> Terminator6/1
  [A] -> Kalman Filter for Pitch/5(newAngle)
  I2C Master Read3/1 -> Data Type Conversion3/1
  Kalman Filter for Roll/2(P_temp) -> Terminator2/1
  [B] -> Kalman Filter for Pitch/6(newRate)
  Constant7/1 -> Kalman Filter for Pitch/2(Q_angle)
  [C] -> Kalman Filter for Roll/5(newAngle)
  Data Type Conversion/1 -> MATLAB Function1/1(gyrRawX)
  Data Type Conversion2/1 -> MATLAB Function1/2(gyrRawY)
  Kalman Filter for Roll/6(rate) -> Terminator1/1
  Constant6/1 -> Kalman Filter for Pitch/4(R)
  Constant8/1 -> Kalman Filter for Pitch/1(dt)
  MATLAB Function2/1(roll) -> Gain/1
  Constant2/1 -> Kalman Filter for Roll/3(Q_bias)
  Constant4/1 -> Kalman Filter for Roll/2(Q_angle)
  I2C Master Read5/1 -> Data Type Conversion5/1
  Kalman Filter for Pitch/4(bias) -> Terminator8/1
  Kalman Filter for Pitch/6(rate) -> Terminator11/1
  Data Type Conversion5/1 -> MATLAB Function/3(accRawZ)
  MATLAB Function1/2(gyrRateY) -> [B], Scope2/1
  Data Type Conversion4/1 -> MATLAB Function/2(accRawY)
  I2C Master Read4/1 -> Data Type Conversion4/1
  Kalman Filter for Roll/5(y) -> Terminator5/1
  Constant1/1 -> Kalman Filter for Pitch/3(Q_bias)
  Constant11/1 -> psi/1

== matlab function amalifuzzypid/PLANT/Subsystem/MATLAB Function2 ==
  data: dt input; roll output; pitch output; gyrRawX input; gyrRawY input; accAngleX input; accAngleY input
function [roll, pitch] = complimentaryF(dt, gyrRawX, gyrRawY, accAngleX, accAngleY)

 gyrAngleX = gyrRawX * dt;
 gyrAngleY = gyrRawY * dt;
 roll = 0.98 * (gyrAngleX) + 0.02 * accAngleX;
 pitch = 0.98 * (gyrAngleY) + 0.02 * accAngleY;
 
end

== matlab function amalifuzzypid/MATLAB Function ==
  data: u1 output; e input; phi input; theta input
function u1 = fcn(e,phi,theta)
%#codegen
u1=(e+10)/(cosd(phi)*cosd(theta));

== matlab function amalifuzzypid/PLANT/Subsystem/MATLAB Function ==
  data: accRawX input; accAngleX output; accAngleY output; accRawY input; accRawZ input; accAngleZ output
function [accAngleX, accAngleY, accAngleZ] = fcn(accRawX, accRawY, accRawZ)

%Converting the raw accel data from g values to accel about X and Y axis

accAngleX = atan(accRawY/sqrt(power(accRawX,2) + power(accRawZ,2)))*(180/pi);
accAngleY = atan(-1*(accRawX/sqrt(power(accRawY,2) + power(accRawZ,2))))*(180/pi);
accAngleZ = atan(accRawZ/sqrt(power(accRawX,2) + power(accRawZ,2)))*(180/pi);

end

== matlab function amalifuzzypid/MATLAB Function1 ==
  data: U1 input; w1 output; U2 input; U3 input; U4 input; w2 output; w3 output; w4 output
function [w1,w2,w3,w4] = fcn(U1,U2,U3,U4)

w1=real(sqrt(complex(6733*U1-26932*U3-372023*U4)));
w2=real(sqrt(complex(6733*U1-26932*U2+372023*U4)));
w3=real(sqrt(complex(6733*U1+26932*U3-372023*U4)));
w4=real(sqrt(complex(6733*U1+26932*U2+372023*U4)));
end

== matlab function amalifuzzypid/PLANT/MATLAB Function ==
  data: phi input; xdd output; teta input; psi input; ydd output; zdd output; U1 input
function [xdd,ydd,zdd] = fcn(phi,teta,psi,U1)
%#codegen
xdd=((cos(phi)*sin(teta)*cos(psi))+(sin(phi)*sin(psi)))*U1;
ydd=((cos(phi)*sin(teta)*sin(psi))+(sin(phi)*cos(psi)))*U1;
zdd=-9.81+(cos(phi)*cos(teta)*U1);
end

== matlab function amalifuzzypid/PLANT/Subsystem/MATLAB Function1 ==
  data: gyrRawX input; gyrRateX output; gyrRateY output; gyrRawY input; gyrRawZ input; gyrRateZ output
function [gyrRateX, gyrRateY, gyrRateZ] = fcn(gyrRawX, gyrRawY, gyrRawZ)

gyrRateX = gyrRawX/131.0;
gyrRateY = gyrRawY/131.0;
gyrRateZ = gyrRawZ/131.0;

end

== matlab function amalifuzzypid/PLANT/Subsystem/Kalman Filter for Pitch ==
  data: dt input; pitch output; Q_angle input; Q_bias input; R input; newAngle input; newRate input; P_temp output; K output; bias output; y output; rate output
function [pitch, P_temp, K, bias, y, rate]  = kalFilterPitch(dt, Q_angle, Q_bias, R, newAngle, newRate)

persistent angle;
persistent P;


%Process Noise Convariance Matrix
Q = [Q_angle 0; 0 Q_bias] * dt;
F = [1  dt; 0 1];
H = [1 0];
bias = 6.8186;

rate = newRate - bias;

if isempty(angle); angle = 0;
    
else
    angle = angle + (dt * rate);
end 

pitch = angle;

if isempty(P); P = [0, 0; 0, 0];
else
    P = F*P*F' + Q;
end 
P_temp = P;

S = H*P*H' + R;
K = (P_temp * H')/S;
y = newAngle - pitch; 
pitch = pitch + K(1) * y;
bias = pitch + K(2) * y;
angle = pitch;

I = [1 0; 0 1];
P_temp = (I - K*H)*P_temp;
P = P_temp;

return 


end

== matlab function amalifuzzypid/PLANT/Subsystem/Kalman Filter for Roll ==
  data: dt input; roll output; Q_angle input; Q_bias input; R input; newAngle input; newRate input; P_temp output; K output; bias output; y output; rate output
function [roll, P_temp, K, bias, y, rate]  = kalFilterRoll(dt, Q_angle, Q_bias, R, newAngle, newRate)

persistent angle;
persistent P;


%Process Noise Convariance Matrix
Q = [Q_angle 0; 0 Q_bias] * dt;
F = [1  dt; 0 1];
H = [1 0];
bias = 3.4532;

rate = newRate - bias;

if isempty(angle); angle = 0;
    
else
    angle = angle + (dt * rate);
end 

roll = angle;

if isempty(P); P = [0, 0; 0, 0];
else
    P = F*P*F' + Q;
end 
P_temp = P;

S = H*P*H' + R;
K = (P_temp * H')/S;
y = newAngle - roll; 
roll = roll + K(1) * y;
bias = roll + K(2) * y;
angle = roll;

I = [1 0; 0 1];
P_temp = (I - K*H)*P_temp;
P = P_temp;

return 


end
